simulink model "mpc_controle_modelo"  (R2025a)
settings: Solver=VariableStepAuto  StartTime=0.0  StopTime=350.0  RelTol=1e-3
libraries: cstblocks x1, mpclib x1
settings Model: Creator=joaof  LastModifiedBy=joaof

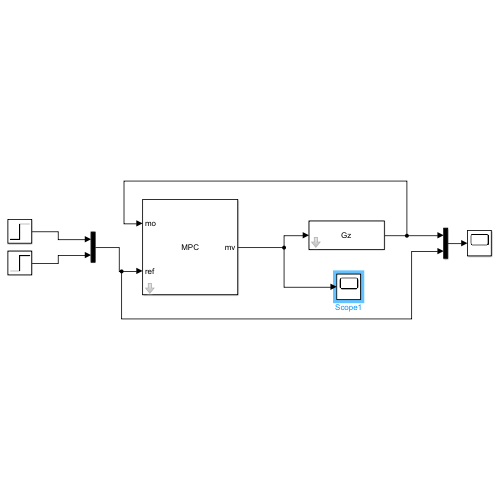
[thumbnail: Simulink's stored preview of the top-level diagram]
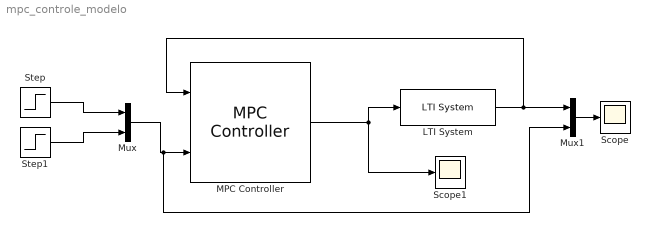
== system mpc_controle_modelo ==
  LTI System : cstblocks/LTI System  sys=Gz  IC=[]  PadeOrder=0
  MPC Controller : mpclib/MPC Controller  SCDEnableBlockLinearizationSpecification=on  mpcobj=mpcobj  is_multiple=0  enable_value=0  return_u0=off  updateMPCinCallerWorkspace=on  md_inport=off  mv_inport=off  uref_inport=off  return_cost=off  return_mvseq=off  return_qpstatus=off  return_xseq=off  return_state=off  return_ovseq=off  state_inport=off  umin_inport=off  umax_inport=off  ymin_inport=off  ymax_inport=off  cc_inport=off  ywt_inport=off  uwt_inport=off  duwt_inport=off  rhoeps_inport=off  pm_inport=off  MaximumP=10  HorizonChoice=FixedHorizon  n_ts=0.1  n_p=20  n_mv=2  n_md=0  n_ud=0  n_mo=2  n_uo=0  BlockDataType=double  SampleTimeInherited=off  switch_inport=off
  Mux : Mux  Inputs=2
  Mux1 : Mux  Inputs=2
  Scope : Scope
      settings: ActiveDisplayYMinimum=-0.0485124915400474  ActiveDisplayYMaximum=0.43661242386042676
  Scope1 : Scope
      settings: ActiveDisplayYMinimum=-1.2499999999999998  ActiveDisplayYMaximum=11.25
  Step : Step  Time=200  Before=0.25  After=0.28  SampleTime=0
  Step1 : Step  Time=200  Before=0.35  After=0.38  SampleTime=0
  wires:
  MPC Controller/1 -> Scope1/1, LTI System/1
  LTI System/1 -> Mux1/1, MPC Controller/1
  Mux/1 -> Mux1/2, MPC Controller/2
  Step/1 -> Mux/1
  Step1/1 -> Mux/2
  Mux1/1 -> Scope/1
